simulink model "PlaneSimulationModel_r17"  (R2022b)
settings: Solver=FixedStepAuto  StartTime=0.0  StopTime=20  FixedStep=0.0025  RelTol=1e-3
values from neighbouring files (symbols this model uses):
  bref = 2.43    [plane_sm_dictionary.sldd]
  cref = 0.2977    [plane_sm_dictionary.sldd]
  g = 9.81    [plane_sm_dictionary.sldd]
  Ix = 0.810078    [plane_sm_dictionary.sldd]
  Iy = 1.177574    [plane_sm_dictionary.sldd]
  Iz = 1.346181    [plane_sm_dictionary.sldd]
  m = 6.67    [plane_sm_dictionary.sldd]
  pochodne = 0.721    [plane_sm_dictionary.sldd]
  Sref = 0.721    [plane_sm_dictionary.sldd]
settings Model: DataDictionary=plane_sm_dictionary.sldd  EnableAccessToBaseWorkspace=off  PauseTimes=0  Creator=Marcin  LastModifiedBy=Wojtek
settings SolverCC: AlgebraicLoopSolver=TrustRegion
settings DataIOCC: ReturnWorkspaceOutputs=off
settings OptimizationCC: DefaultParameterBehavior=Inlined  UseDivisionForNetSlopeComputation=on  DefaultUnderspecifiedDataType=single  PassReuseOutputArgsAs=Individual arguments  EfficientTunableParamExpr=on
settings DebuggingCC: ParameterTunabilityLossMsg=error  UnconnectedInputMsg=warning  UnconnectedOutputMsg=warning  UnconnectedLineMsg=warning  SFMachineParentedDataDiag=warning  ArithmeticOperatorsInVariantConditions=warning
settings HardwareCC: ProdBitPerPointer=32  ProdBitPerSizeT=32  ProdBitPerPtrDiffT=32  ProdLargestAtomicInteger=Long  ProdLargestAtomicFloat=Double  ProdWordSize=32  ProdHWDeviceType=ARM Compatible->ARM Cortex-M
settings ModelReferenceCC: EnableRefExpFcnMdlSchedulingChecks=on
settings SFSimCC: SimUseLocalCustomCode=off  MATLABDynamicMemAlloc=off  CustomCodeUndefinedFunction=UseInterfaceOnly
settings RTWCC: Description=Embedded Coder  SystemTargetFile=ert.tlc  TemplateMakefile=ert_default_tmf  GenerateReport=on  RTWUseLocalCustomCode=off  Toolchain=MinGW64 | gmake (64-bit Windows)  IncludeHyperlinkInReport=on  LaunchReport=on  GenerateTraceInfo=on  GenerateTraceReport=on  GenerateTraceReportSl=on  GenerateTraceReportSf=on  GenerateTraceReportEml=on
settings CodeAppCC: ForceParamTrailComments=on  OperatorAnnotations=on  SimulinkDataObjDesc=on  SFDataObjDesc=on  InsertBlockDesc=on
settings ERTTargetCC: TargetLangStandard=C99 (ISO)  CodeReplacementLibrary=GNU C99 extensions  SupportVariableSizeSignals=on  InlinedParameterPlacement=NonHierarchical  ERTCustomFileTemplate=example_file_process.tlc  MemSecPackage=Simulink

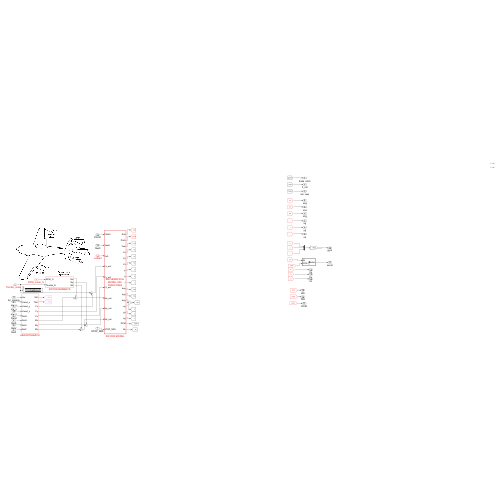
[thumbnail: Simulink's stored preview of the top-level diagram]
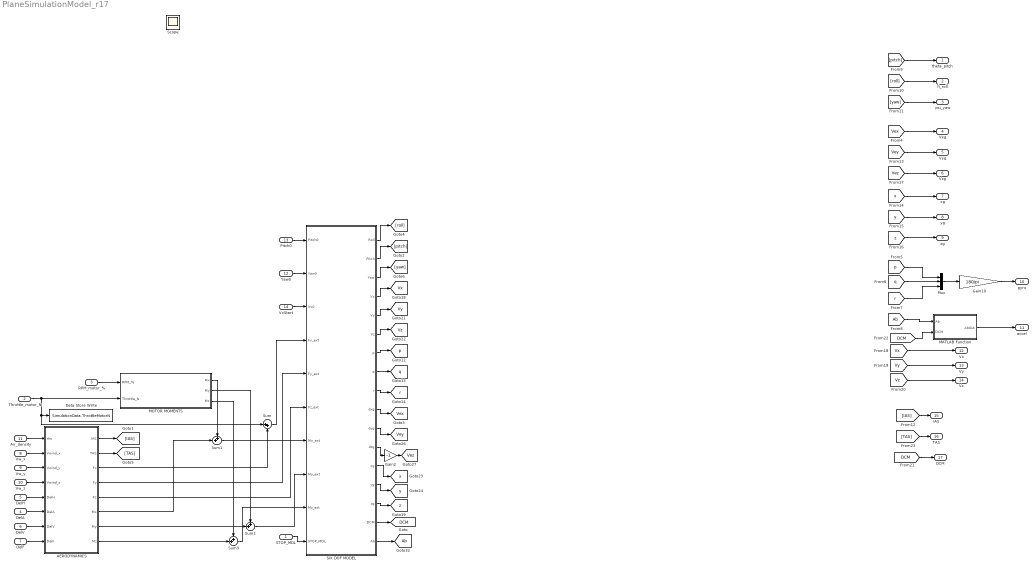
== system PlaneSimulationModel_r17 ==
  STOP_MDL : Inport  OutDataTypeStr=boolean
  Throttle_motor_N : Inport  Port=2  OutDataTypeStr=double
  RPM_motor_% : Inport  Port=3  OutDataTypeStr=double
  DelA : Inport  Port=4  OutDataTypeStr=double
  DelH : Inport  Port=5  OutDataTypeStr=double
  DelV : Inport  Port=6  OutDataTypeStr=double
  DelF : Inport  Port=7  OutDataTypeStr=double
  Vw_x : Inport  Port=8  OutDataTypeStr=double
  Vw_y : Inport  Port=9  OutDataTypeStr=double
  Vw_z : Inport  Port=10  OutDataTypeStr=double
  Air_density : Inport  Port=11  OutDataTypeStr=double
  Yaw0 : Inport  Port=12  OutDataTypeStr=double
  Pitch0 : Inport  Port=13  OutDataTypeStr=double
  VxStart : Inport  Port=14  OutDataTypeStr=double
  AERODYNAMICS : Subsystem
  Data Store Write : DataStoreWrite  DataStoreName=SimulationData  DataStoreElements=SimulationData.ThrottleMotorN  IndexOptions=Index vector (dialog)  Indices=1  OutputSizes=1
  Gain10 : Gain  Gain=180/pi
  Gain2 : Gain  Gain=-1
  MATLAB Function : MATLAB Function  TreatAsAtomicUnit=on
  MOTOR MOMENTS : Subsystem
  Mux : Mux  Inputs=3
  SIX DOF MODEL : MATLAB Function  Priority=0  TreatAsAtomicUnit=on  SystemSampleTime=0.0025
  Sum : Sum  Inputs=|++
  Sum1 : Sum  Inputs=++|
  Sum2 : Sum  Inputs=++|
  Sum3 : Sum  Inputs=++|
  theta_pitch : Outport  VectorParamsAs1DForOutWhenUnconnected=off
  fi_roll : Outport  Port=2  VectorParamsAs1DForOutWhenUnconnected=off
  psi_yaw : Outport  Port=3  VectorParamsAs1DForOutWhenUnconnected=off
  Vxg : Outport  Port=4  VectorParamsAs1DForOutWhenUnconnected=off
  Vyg : Outport  Port=5  VectorParamsAs1DForOutWhenUnconnected=off
  Vzg : Outport  Port=6  VectorParamsAs1DForOutWhenUnconnected=off
  xg : Outport  Port=7  VectorParamsAs1DForOutWhenUnconnected=off
  yg : Outport  Port=8  VectorParamsAs1DForOutWhenUnconnected=off
  zg : Outport  Port=9  VectorParamsAs1DForOutWhenUnconnected=off
  gyro : Outport  Port=10  VectorParamsAs1DForOutWhenUnconnected=off
  accel : Outport  Port=11  VectorParamsAs1DForOutWhenUnconnected=off
  Vx : Outport  Port=12  VectorParamsAs1DForOutWhenUnconnected=off
  Vy : Outport  Port=13  VectorParamsAs1DForOutWhenUnconnected=off
  Vz : Outport  Port=14  VectorParamsAs1DForOutWhenUnconnected=off
  IAS : Outport  Port=15  OutDataTypeStr=double  VectorParamsAs1DForOutWhenUnconnected=off
  TAS : Outport  Port=16  OutDataTypeStr=double  VectorParamsAs1DForOutWhenUnconnected=off
  DCM : Outport  Port=17  OutDataTypeStr=double  VectorParamsAs1DForOutWhenUnconnected=off
  Scope : Scope
  tag scope: Ab=global, DCM=global, Vex=global, Vey=global, Vez=global, Vx=global, Vy=global, Vz=global, p=global, q=global, r=global, x=global, y=global, z=global
  wires:
  SIX DOF MODEL/15(zg) -> [z]
  SIX DOF MODEL/16(DCM) -> [DCM]
  Gain2/1 -> [Vez]
  SIX DOF MODEL/13(xg) -> [x]
  SIX DOF MODEL/14(yg) -> [y]
  SIX DOF MODEL/17(Ab) -> [Ab]
  STOP_MDL/1 -> SIX DOF MODEL/10(STOP_MDL)
  ? -> ?
  ? -> ?
  [pitch] -> theta_pitch/1
  Mux/1 -> Gain10/1
  [yaw] -> psi_yaw/1
  [roll] -> fi_roll/1
  [IAS] -> IAS/1
  [r] -> Mux/3
  [q] -> Mux/2
  [p] -> Mux/1
  [y] -> yg/1
  [z] -> zg/1
  [x] -> xg/1
  Throttle_motor_N/1 -> MOTOR MOMENTS/2(Throttle_N), Data Store Write/1, Sum/1
  Air_density/1 -> AERODYNAMICS/1(rho)
  Vw_x/1 -> AERODYNAMICS/2(Vwind_x)
  Vw_y/1 -> AERODYNAMICS/3(Vwind_y)
  Vw_z/1 -> AERODYNAMICS/4(Vwind_z)
  DelH/1 -> AERODYNAMICS/5(DelH)
  DelA/1 -> AERODYNAMICS/6(DelA)
  DelV/1 -> AERODYNAMICS/7(DelV)
  DelF/1 -> AERODYNAMICS/8(DelF)
  AERODYNAMICS/3(Fx) -> Sum/2
  AERODYNAMICS/1(IAS) -> [IAS]
  AERODYNAMICS/4(Fy) -> SIX DOF MODEL/5(Fy_ext)
  AERODYNAMICS/5(Fz) -> SIX DOF MODEL/6(Fz_ext)
  [Vex] -> Vxg/1
  [Vey] -> Vyg/1
  [Vez] -> Vzg/1
  [Vx] -> Vx/1
  [Vy] -> Vy/1
  [Vz] -> Vz/1
  Gain10/1 -> gyro/1
  RPM_motor_%/1 -> MOTOR MOMENTS/1(RPM_%)
  AERODYNAMICS/6(Mx) -> Sum1/2
  Sum1/1 -> SIX DOF MODEL/7(Mx_ext)
  AERODYNAMICS/7(My) -> Sum2/2
  AERODYNAMICS/8(Mz) -> Sum3/2
  Sum3/1 -> SIX DOF MODEL/9(Mz_ext)
  Sum2/1 -> SIX DOF MODEL/8(My_ext)
  MOTOR MOMENTS/1(Mx) -> Sum1/1
  MOTOR MOMENTS/2(My) -> Sum2/1
  MOTOR MOMENTS/3(Mz) -> Sum3/1
  [DCM] -> DCM/1
  MATLAB Function/1(AbOut) -> accel/1
  [Ab] -> MATLAB Function/1(Ab)
  [DCM] -> MATLAB Function/2(DCM)
  AERODYNAMICS/2(TAS) -> [TAS]
  [TAS] -> TAS/1
  VxStart/1 -> SIX DOF MODEL/3(Vx0)
  Yaw0/1 -> SIX DOF MODEL/2(Yaw0)
  Pitch0/1 -> SIX DOF MODEL/1(Pitch0)
  SIX DOF MODEL/12(dzg) -> Gain2/1
  SIX DOF MODEL/10(dxg) -> [Vex]
  SIX DOF MODEL/11(dyg) -> [Vey]
  SIX DOF MODEL/6(Vz) -> [Vz]
  SIX DOF MODEL/5(Vy) -> [Vy]
  SIX DOF MODEL/4(Vx) -> [Vx]
  SIX DOF MODEL/7(p) -> [p]
  SIX DOF MODEL/8(q) -> [q]
  SIX DOF MODEL/9(r) -> [r]
  SIX DOF MODEL/2(Pitch) -> [pitch]
  SIX DOF MODEL/1(Roll) -> [roll]
  SIX DOF MODEL/3(Yaw) -> [yaw]
  Sum/1 -> SIX DOF MODEL/4(Fx_ext)

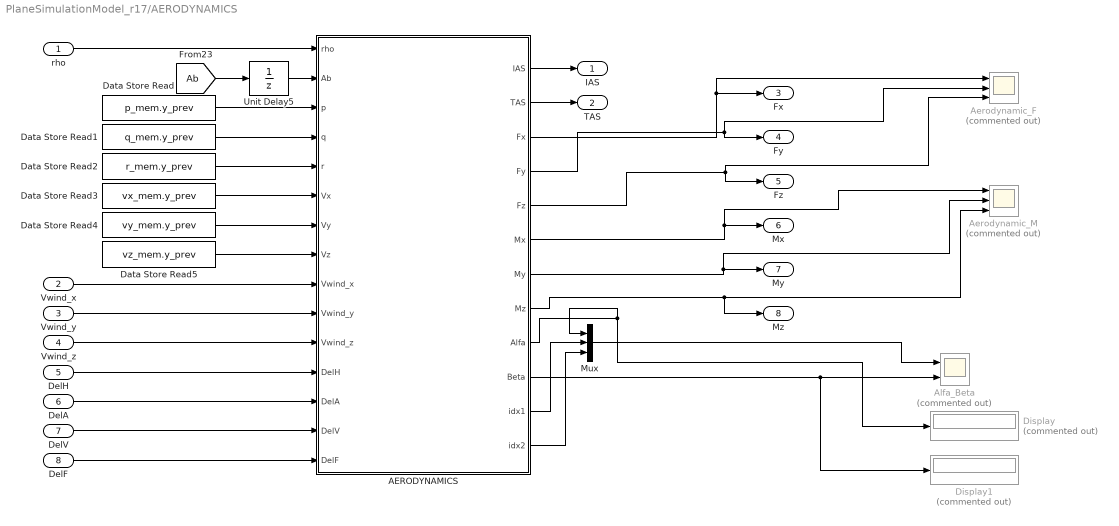
== system PlaneSimulationModel_r17/AERODYNAMICS ==
  rho : Inport
  Vwind_x : Inport  Port=2
  Vwind_y : Inport  Port=3
  Vwind_z : Inport  Port=4
  DelH : Inport  Port=5
  DelA : Inport  Port=6
  DelV : Inport  Port=7
  DelF : Inport  Port=8
  AERODYNAMICS : MATLAB Function  TreatAsAtomicUnit=on
  Aerodynamic_F : Scope  Commented=on  NumInputPorts=3
  Aerodynamic_M : Scope  Commented=on  NumInputPorts=3
  Alfa_Beta : Scope  Commented=on  NumInputPorts=2
  Data Store Read : DataStoreRead  DataStoreName=p_mem  DataStoreElements=p_mem.y_prev  IndexOptions=Index vector (dialog)  Indices=1  OutputSizes=1
  Data Store Read1 : DataStoreRead  DataStoreName=q_mem  DataStoreElements=q_mem.y_prev  IndexOptions=Index vector (dialog)  Indices=1  OutputSizes=1
  Data Store Read2 : DataStoreRead  DataStoreName=r_mem  DataStoreElements=r_mem.y_prev  IndexOptions=Index vector (dialog)  Indices=1  OutputSizes=1
  Data Store Read3 : DataStoreRead  DataStoreName=vx_mem  DataStoreElements=vx_mem.y_prev  IndexOptions=Index vector (dialog)  Indices=1  OutputSizes=1
  Data Store Read4 : DataStoreRead  DataStoreName=vy_mem  DataStoreElements=vy_mem.y_prev  IndexOptions=Index vector (dialog)  Indices=1  OutputSizes=1
  Data Store Read5 : DataStoreRead  DataStoreName=vz_mem  DataStoreElements=vz_mem.y_prev  IndexOptions=Index vector (dialog)  Indices=1  OutputSizes=1
  Display : Display  Commented=on
  Display1 : Display  Commented=on
  Mux : Mux  Inputs=3
  Unit Delay5 : UnitDelay  SampleTime=-1  HasFrameUpgradeWarning=on
  IAS : Outport
  TAS : Outport  Port=2
  Fx : Outport  Port=3
  Fy : Outport  Port=4
  Fz : Outport  Port=5
  Mx : Outport  Port=6
  My : Outport  Port=7
  Mz : Outport  Port=8
  wires:
  DelF/1 -> AERODYNAMICS/15(DelF)
  Data Store Read1/1 -> AERODYNAMICS/4(q)
  AERODYNAMICS/8(Mz) -> Mz/1, Aerodynamic_M/3
  DelH/1 -> AERODYNAMICS/12(DelH)
  Data Store Read/1 -> AERODYNAMICS/3(p)
  Data Store Read5/1 -> AERODYNAMICS/8(Vz)
  Data Store Read4/1 -> AERODYNAMICS/7(Vy)
  Data Store Read3/1 -> AERODYNAMICS/6(Vx)
  Data Store Read2/1 -> AERODYNAMICS/5(r)
  AERODYNAMICS/6(Mx) -> Aerodynamic_M/1, Mx/1
  DelV/1 -> AERODYNAMICS/14(DelV)
  rho/1 -> AERODYNAMICS/1(rho)
  AERODYNAMICS/3(Fx) -> Aerodynamic_F/1, Fx/1
  Vwind_x/1 -> AERODYNAMICS/9(Vwind_x)
  Vwind_y/1 -> AERODYNAMICS/10(Vwind_y)
  AERODYNAMICS/5(Fz) -> Aerodynamic_F/3, Fz/1
  Vwind_z/1 -> AERODYNAMICS/11(Vwind_z)
  DelA/1 -> AERODYNAMICS/13(DelA)
  AERODYNAMICS/7(My) -> Aerodynamic_M/2, My/1
  AERODYNAMICS/4(Fy) -> Aerodynamic_F/2, Fy/1
  AERODYNAMICS/1(IAS) -> IAS/1
  AERODYNAMICS/9(Alfa) -> Mux/1, Display/1
  AERODYNAMICS/10(Beta) -> Display1/1, Alfa_Beta/2
  Mux/1 -> Alfa_Beta/1
  AERODYNAMICS/12(idx2) -> Mux/3
  AERODYNAMICS/11(idx1) -> Mux/2
  [Ab] -> Unit Delay5/1
  Unit Delay5/1 -> AERODYNAMICS/2(Ab)
  AERODYNAMICS/2(TAS) -> TAS/1

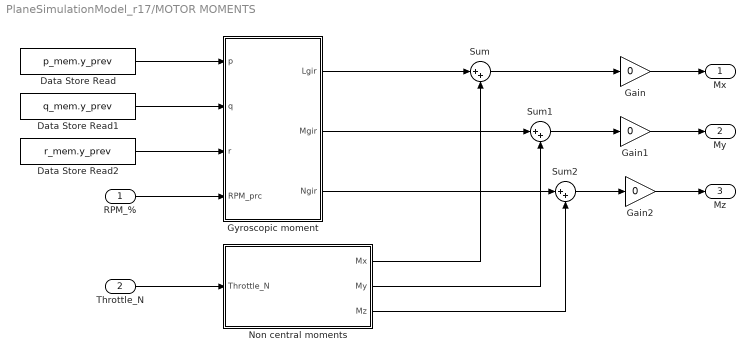
== system PlaneSimulationModel_r17/MOTOR MOMENTS ==
  RPM_% : Inport
  Throttle_N : Inport  Port=2
  Data Store Read : DataStoreRead  DataStoreName=p_mem  DataStoreElements=p_mem.y_prev  IndexOptions=Index vector (dialog)  Indices=1  OutputSizes=1
  Data Store Read1 : DataStoreRead  DataStoreName=q_mem  DataStoreElements=q_mem.y_prev  IndexOptions=Index vector (dialog)  Indices=1  OutputSizes=1
  Data Store Read2 : DataStoreRead  DataStoreName=r_mem  DataStoreElements=r_mem.y_prev  IndexOptions=Index vector (dialog)  Indices=1  OutputSizes=1
  Gain : Gain  Gain=0
  Gain1 : Gain  Gain=0
  Gain2 : Gain  Gain=0
  Gyroscopic moment : MATLAB Function  TreatAsAtomicUnit=on
  Non central moments : MATLAB Function  TreatAsAtomicUnit=on
  Sum : Sum  Inputs=|++
  Sum1 : Sum  Inputs=|++
  Sum2 : Sum  Inputs=|++
  Mx : Outport
  My : Outport  Port=2
  Mz : Outport  Port=3
  wires:
  Throttle_N/1 -> Non central moments/1(Throttle_N)
  Data Store Read2/1 -> Gyroscopic moment/3(r)
  Data Store Read1/1 -> Gyroscopic moment/2(q)
  Data Store Read/1 -> Gyroscopic moment/1(p)
  RPM_%/1 -> Gyroscopic moment/4(RPM_prc)
  Sum/1 -> Gain/1
  Gyroscopic moment/1(Lgir) -> Sum/1
  Sum1/1 -> Gain1/1
  Non central moments/2(My) -> Sum1/2
  Gyroscopic moment/2(Mgir) -> Sum1/1
  Sum2/1 -> Gain2/1
  Gyroscopic moment/3(Ngir) -> Sum2/1
  Non central moments/3(Mz) -> Sum2/2
  Non central moments/1(Mx) -> Sum/2
  Gain/1 -> Mx/1
  Gain1/1 -> My/1
  Gain2/1 -> Mz/1

== matlab function PlaneSimulationModel_r17/AERODYNAMICS/AERODYNAMICS ==
  data: rho input; Ab input; p input; q input; r input; Vx input; Vy input; Vz input; IAS output size=1; TAS output size=1; Vwind_x input; Fx output size=1; Fy output size=1; Fz output size=1; Mx output size=1; My output size=1; Mz output size=1; Vwind_y input; Vwind_z input; DelH input; DelA input; DelV input; DelF input; Ix parameter; Iy parameter; Iz parameter; g parameter; m parameter; pochodne parameter; cref parameter; bref parameter; Sref parameter; Alfa output size=1; Beta output size=1; idx1 output size=1; idx2 output size=1; SimulationData data_store_memory
function [IAS, TAS,Fx,Fy,Fz,Mx,My,Mz,Alfa,Beta,idx1,idx2]= fcn(rho,Ab,p,q,r,Vx,Vy,Vz,Vwind_x,Vwind_y,Vwind_z,DelH,DelA,DelV,DelF, Ix, Iy, Iz, g, m, pochodne, cref, bref, Sref)

global SimulationData

persistent alfa; if isempty(alfa) alfa = double(0);end
persistent alfa_old; if isempty(alfa_old) alfa_old = double(0);end
persistent beta; if isempty(beta) beta = double(0);end

    sa = sin(alfa);
    sb = sin(beta);
    ca = cos(alfa);
    cb = cos(beta);    

    %% Transition matrix from the flow-related system to the object-related system

    Lba = [ca*cb      -ca*sb      -sa;...
            sb         cb           0;...
           sa*cb      -sa*sb      ca]; 

    %% Taking into account the wind speed in the system related to the object
   
    Vaer_x = Vx - Vwind_x;
    Vaer_y = Vy - Vwind_y;
    Vaer_z = Vz - Vwind_z;
    
    TAS = sqrt(Vaer_x^2+Vaer_y^2+Vaer_z^2);%modul predkosci aerodynamicznej
    rho0 = double(1.225);
    IAS = TAS*sqrt(rho/rho0);
 
 %% Wyznaczenie kąta natarcia i ślizgu aerodynamicznych
    if(Vaer_x ~= 0)
        alfa = atan(Vaer_z / Vaer_x); 
    else
        alfa = double(0);
    end
        
    if(TAS ~= 0) 
        beta = asin(Vaer_y / TAS);
    else
        beta = double(0);
    end
    
   
    Alfa = alfa*180/pi;
    Beta = beta*180/pi;


    [idx1,idx2] = FindClosestAlfa(pochodne.Alfa, Alfa);

    Cxa = CDa_from_table(pochodne,idx1,idx2,Alfa,DelH,DelF,q,cref,TAS);
    Cy = Cy_from_table(pochodne,idx1,idx2,Alfa,Beta,DelA,DelV,p,r,bref,TAS);
    Cza = CLa_from_table(pochodne,idx1,idx2,Alfa,DelH,DelF,q,cref,TAS, 0);

    
    Q=rho*TAS^2/2; 
    % resistance force
    Rxa = -Cxa*Q*Sref;
    % lifting force
    Rza = -Cza*Q*Sref; 

    temp_Rxyz= Lba*[Rxa;0;Rza];
   
    
    Fx=temp_Rxyz(1);
    Fy=temp_Rxyz(2) + Cy*Q*Sref;
    Fz=temp_Rxyz(3);

    
    %% Determining moments acting on an object in the xyz coordinate system
    %% Aerodynamic moments
    Cl = Cl_from_table(pochodne,idx1,idx2,Alfa,Beta,DelA,DelV,p,r,bref,TAS);
    Cm = Cm_from_table(pochodne,idx1,idx2,Alfa,DelH,DelF,q,cref,TAS,Ab(3)); 
    Cn = Cn_from_table(pochodne,idx1,idx2,Alfa,Beta,DelA,DelV,p,r,bref,TAS);

    Mx = Cl*Q*bref*Sref;
    My = Cm*Q*cref*Sref;
    Mz = Cn*Q*bref*Sref;



    SimulationData.rho = rho;
    SimulationData.IAS = IAS;
    SimulationData.Cxa = Cxa;
    SimulationData.Cy = Cy;
    SimulationData.Cza = Cza;
    SimulationData.Fx = Fx;
    SimulationData.Fy = Fy;
    SimulationData.Fz = Fz;
    SimulationData.Cl = Cl;
    SimulationData.Cm = Cm;
    SimulationData.Cn = Cn;
    SimulationData.Mx = Mx;
    SimulationData.My = My;
    SimulationData.Mz = Mz;

    SimulationData.Alfa = Alfa;
    SimulationData.Beta = Beta;

    SimulationData.p = p;
    SimulationData.q = q;
    SimulationData.r = r;
    SimulationData.DelH = DelH;
    SimulationData.DelA = DelA;
    SimulationData.DelV = DelV;
    SimulationData.DelF = DelF;

== matlab function PlaneSimulationModel_r17/MOTOR MOMENTS/Non central moments ==
  data: Throttle_N input; Mx output; My output; Mz output
function [Mx,My,Mz]= fcn(Throttle_N)
% z offset in body cordinates
z_offset = 0;

Mx = 0;
My = Throttle_N * z_offset;
Mz = 0;

== matlab function PlaneSimulationModel_r17/MOTOR MOMENTS/Gyroscopic moment ==
  data: p input; Lgir output; q input; r input; RPM_prc input; Mgir output; Ngir output
function [Lgir,Mgir,Ngir] = fcn(p,q,r,RPM_prc)
Kp = 0.01;
J = 0.001;
omega_x = RPM_prc*Kp; 
omega_y = 0;
omega_z = 0;
Lgir=J*(sum(omega_y)*r-sum(omega_z)*q);
Mgir=J*(sum(omega_z)*p-sum(omega_x)*r);
Ngir=J*(sum(omega_x)*q-sum(omega_y)*p);

== matlab function PlaneSimulationModel_r17/MATLAB Function ==
  data: Ab input; AbOut output; DCM input; g parameter
function AbOut = fcn(Ab, DCM, g)



AbOut =  Ab + DCM' * [0; 0; -g];

== matlab function PlaneSimulationModel_r17/SIX DOF MODEL ==
  settings: updateMethod=DISCRETE
  data: Pitch0 input; Yaw0 input; Vx0 input; m parameter; Ix parameter; Iy parameter; Iz parameter; g parameter; Fx_ext input; Fy_ext input; Fz_ext input; Mx_ext input; My_ext input; Mz_ext input; STOP_MDL input; Roll output double; Pitch output double; Yaw output double; Vx output double; Vy output double; Vz output double; p output double; q output double; r output double; dxg output double; dyg output double; dzg output double; xg output; yg output; zg output; DCM output double; Ab output double size=[3 1]; p_mem data_store_memory; q_mem data_store_memory; r_mem data_store_memory; vx_mem data_store_memory; vy_mem data_store_memory; vz_mem data_store_memory; roll_mem data_store_memory; pitch_mem data_store_memory; yaw_mem data_store_memory; xg_mem data_store_memory; yg_mem data_store_memory; zg_mem data_store_memory
function [Roll, Pitch, Yaw, ... speed of change of angles 
          Vx, Vy, Vz, ... linear accelerations
          p, q, r, ... rotational accelerations
          dxg,dyg,dzg, ... velocities in the earth-related system
          xg,yg,zg,...
          DCM, ... z q do g
          Ab]... acceleration of the object
          = fcn(Pitch0,Yaw0,Vx0,...         
          m,Ix, Iy, Iz,...
          g,...
          Fx_ext,Fy_ext,Fz_ext,...
          Mx_ext,My_ext,Mz_ext,STOP_MDL)...)...
%#codegen

%% 
global p_mem q_mem r_mem
global roll_mem pitch_mem yaw_mem
global vx_mem vy_mem vz_mem
global xg_mem yg_mem zg_mem

persistent init; if isempty(init); init = false;end

if(init == false)
    
    pitch_mem.y_prev = Pitch0;
    yaw_mem.y_prev = Yaw0;
    vx_mem.y_prev = Vx0;
    
    init = true;

end

dt=0.0025;


%% assign local variables from memory
p = p_mem.y_prev;
q = q_mem.y_prev;
r = r_mem.y_prev;

Roll = wrap_180(roll_mem.y_prev*180/pi);
Pitch = wrap_180(pitch_mem.y_prev*180/pi);
Yaw = wrap_180(yaw_mem.y_prev*180/pi);

Vx = vx_mem.y_prev;
Vy = vy_mem.y_prev;
Vz = vz_mem.y_prev;

xg = xg_mem.y_prev;
yg = yg_mem.y_prev;
zg = zg_mem.y_prev;

%%

if(STOP_MDL)
    init = false;
    sp = sin(0);
    sr = sin(0);
    sy = sin(0);
    cp = cos(0);
    cr = cos(0);
    cy = cos(0);

    %Transition matrix from the inertial frame (bound to the Earth) to the frame
    %bound to the object for the initial conditions
    Lbg = [cy*cp              sy*cp               -sp;...
           cy*sp*sr-sy*cr     sy*sp*sr+cy*cr      cp*sr;...
           cy*sp*cr+sy*sr     sy*sp*cr-cy*sr      cp*cr];
    %Transition matrix from the frame associated with the object to the inertial frame (associated with the Earth)
    Lgb = Lbg'; 
    DCM = Lgb;

    % outputs
    dRoll = double(0);
    dPitch  = double(0);
    dYaw  = double(0);
    dVx  = double(0);
    dVy  = double(0);
    dVz  = double(0);
    dp  = double(0);
    dq  = double(0);
    dr  = double(0);
    dxg = double(0);
    dyg  = double(0);
    dzg  = double(0);
    Ab = double([0; 0; 0]);

    return;
end


    %% Calculation of sines and cosines used in transition matrices
    sp = sin(pitch_mem.y_prev);
    sr = sin(roll_mem.y_prev);
    sy = sin(yaw_mem.y_prev);
    cp = cos(pitch_mem.y_prev);
    cr = cos(roll_mem.y_prev);
    cy = cos(yaw_mem.y_prev);

   

    %% Transition matrices

    %Transition matrix from the inertial frame (related to the Earth) to the frame related to the object
    Lbg=[cy*cp              sy*cp               -sp;...
         cy*sp*sr-sy*cr     sy*sp*sr+cy*cr      cp*sr;...
         cy*sp*cr+sy*sr     sy*sp*cr-cy*sr      cp*cr];
    %Transition matrix from the frame associated with the object to the inertial frame (associated with the Earth)
    Lgb = Lbg'; 
    DCM = Lgb;
  
  
    %% Determination of forces acting on an object in the xyz coordinate system

    %% uwzglednienie sily ciezkosci
    temp_Qxyz = Lbg * [0; 0; m*g];
    Qx = temp_Qxyz(1);
    Qy = temp_Qxyz(2);
    Qz = temp_Qxyz(3);


    %% Resultant moments and forces on individual x, y, z axes in the system related to the object
    Fx = Qx+Fx_ext;
    Fy = Qy+Fy_ext;
    Fz = Qz+Fz_ext;
    Mx = Mx_ext;
    My = My_ext;
    Mz = Mz_ext;
 
    %% Differential equations describing motion in 6 axes
    
    %angular accelerations according to the principle of conservation of rotation/momentum
    dp=(Mx-(Iz-Iy)*q*r)/Ix;
    dq=(My-(Ix-Iz)*p*r)/Iy;
    dr=((Mz -(Iy-Ix)*p*q))/Iz;

    %velocities of changes of angles - kinematic relationships
    dRoll=p+(q*sr+r*cr)*sp/cp;
    dPitch=q*cr-r*sr;
    dYaw=(r*cr+q*sr)/cp;
    
  
    %linear accelerations according to Newton's law of motion
   
    Axb = 1/m*Fx;
    Ayb = 1/m*Fy;
    Azb = 1/m*Fz;
    dVx = Axb + r*Vy-q*Vz;
    dVy = Ayb + p*Vz-r*Vx;
    dVz = Azb + q*Vx-p*Vy;
    %determination of accelerations measured by the accelerometer
    Ab = [Axb;Ayb;Azb];
    
    %determining the velocity in the earth-related system
    [temp_poz_g]=Lgb*[Vx;Vy;Vz];
    dxg=temp_poz_g(1);
    dyg=temp_poz_g(2);
    dzg=temp_poz_g(3);

    %% integration process
    p_mem = trapezoidalIntegrator(dp,dt,p_mem);
    q_mem = trapezoidalIntegrator(dq,dt,q_mem);
    r_mem = trapezoidalIntegrator(dr,dt,r_mem);

    roll_mem = trapezoidalIntegrator(dRoll,dt,roll_mem);
    pitch_mem = trapezoidalIntegrator(dPitch,dt,pitch_mem);
    yaw_mem = trapezoidalIntegrator(dYaw,dt,yaw_mem);

    vx_mem = trapezoidalIntegrator(dVx,dt,vx_mem);
    vy_mem = trapezoidalIntegrator(dVy,dt,vy_mem);
    vz_mem = trapezoidalIntegrator(dVz,dt,vz_mem);

    xg_mem = trapezoidalIntegrator(dVx,dt,xg_mem);
    yg_mem = trapezoidalIntegrator(dVy,dt,yg_mem);
    zg_mem = trapezoidalIntegrator(dVz,dt,zg_mem);

end

function [memory] = trapezoidalIntegrator(u, dt, memory)
% Trapezoidal integrator with fixed time step
% u      - current input value
% dt     - fixed time step
% memory - persistent structure (optionally with initial field y_prev)
%
% y      - integration result
% memory - updated persistent structure

    % Initialize memory if this is the first step
    if isempty(memory) || ~isfield(memory, 'u_prev')
        memory.u_prev = u;

        % If no initial value is provided, assume zero
        if ~isfield(memory, 'y_prev')
            memory.y_prev = 0;
        end

        y = memory.y_prev;
        return;
    end

    % Trapezoidal integration step
    avg_u = 0.5 * (u + memory.u_prev);
    y = memory.y_prev + avg_u * dt;

    % Update memory
    memory.u_prev = u;
    memory.y_prev = y;
end
